simulink model "Pokus07_Display"  (Simulink 8.1)
settings: Solver=ode45  StartTime=0.0  StopTime=10.0  RelTol=1e-3
undefined symbols (not defined in the file): A, ARROW_DOWN, ARROW_LEFT, ARROW_RIGHT, ARROW_UP, ASTERISK, B, BACKSLASH, C, COLON, COMMA, CROSS, CURSOR, D, DOT, ending_column_index, ending_row_index, EQUAL, EXCLAMATION_MARK, F, framebuffer, G, GREATER_THAN, H, HEIGHT, hot, I, J, K, L, LEFT_PARENTHESES, LESS_THAN, M, MINUS, N, O, P, PERCENT, PLUS, POS_X, POS_Y, Q, QUESTION_MARK, QUOTE, R, RECTANGLE, RIGHT_PARENTHESES, S, SEMICOLON, SHARP, SLASH, SPACE, starting_column_index, starting_row_index, T, U, UNDERSCORE, V, W, WIDTH ... (+6)
libraries: dspmtrx3 x197, Common_Library x69, commutil2 x53, simulink_extras x1, dspsnks4 x1
(part 6 of 6)

== system Pokus07_Display/Character_Table/Characters(Q..ARROW_UP)/Char_GREATER_THAN ==
  Byte_01 : Constant  Value=char(:, 2, GREATER_THAN)  OutDataTypeStr=uint8
  Byte_02 : Constant  Value=char(:, 3, GREATER_THAN)  OutDataTypeStr=uint8
  Byte_03 : Constant  Value=char(:, 4, GREATER_THAN)  OutDataTypeStr=uint8
  Byte_04 : Constant  Value=char(:, 5, GREATER_THAN)  OutDataTypeStr=uint8
  Byte_05 : Constant  Value=char(:, 6, GREATER_THAN)  OutDataTypeStr=uint8
  Byte_06 : Constant  Value=char(:, 7, GREATER_THAN)  OutDataTypeStr=uint8
  Byte_07 : Constant  Value=char(:, 8, GREATER_THAN)  OutDataTypeStr=uint8
  Byte_1 : Constant  Value=char(:, 1, GREATER_THAN)  OutDataTypeStr=uint8
  Column_1(1B) : Outport
  Column_2(1B) : Outport  Port=2
  Column_3(1B) : Outport  Port=3
  Column_4(1B) : Outport  Port=4
  Column_5(1B) : Outport  Port=5
  Column_6(1B) : Outport  Port=6
  Column_7(1B) : Outport  Port=7
  Column_8(1B) : Outport  Port=8
  wires:
  Byte_05/1 -> Column_6(1B)/1
  Byte_04/1 -> Column_5(1B)/1
  Byte_01/1 -> Column_2(1B)/1
  Byte_07/1 -> Column_8(1B)/1
  Byte_03/1 -> Column_4(1B)/1
  Byte_06/1 -> Column_7(1B)/1
  Byte_1/1 -> Column_1(1B)/1
  Byte_02/1 -> Column_3(1B)/1

== system Pokus07_Display/Character_Table/Characters(Q..ARROW_UP)/Char_LESS_THAN ==
  Byte_01 : Constant  Value=char(:, 2, LESS_THAN)  OutDataTypeStr=uint8
  Byte_02 : Constant  Value=char(:, 3, LESS_THAN)  OutDataTypeStr=uint8
  Byte_03 : Constant  Value=char(:, 4, LESS_THAN)  OutDataTypeStr=uint8
  Byte_04 : Constant  Value=char(:, 5, LESS_THAN)  OutDataTypeStr=uint8
  Byte_05 : Constant  Value=char(:, 6, LESS_THAN)  OutDataTypeStr=uint8
  Byte_06 : Constant  Value=char(:, 7, LESS_THAN)  OutDataTypeStr=uint8
  Byte_07 : Constant  Value=char(:, 8, LESS_THAN)  OutDataTypeStr=uint8
  Byte_1 : Constant  Value=char(:, 1, LESS_THAN)  OutDataTypeStr=uint8
  Column_1(1B) : Outport
  Column_2(1B) : Outport  Port=2
  Column_3(1B) : Outport  Port=3
  Column_4(1B) : Outport  Port=4
  Column_5(1B) : Outport  Port=5
  Column_6(1B) : Outport  Port=6
  Column_7(1B) : Outport  Port=7
  Column_8(1B) : Outport  Port=8
  wires:
  Byte_05/1 -> Column_6(1B)/1
  Byte_04/1 -> Column_5(1B)/1
  Byte_01/1 -> Column_2(1B)/1
  Byte_07/1 -> Column_8(1B)/1
  Byte_03/1 -> Column_4(1B)/1
  Byte_06/1 -> Column_7(1B)/1
  Byte_1/1 -> Column_1(1B)/1
  Byte_02/1 -> Column_3(1B)/1

== system Pokus07_Display/Character_Table/Characters(Q..ARROW_UP)/Char_MINUS ==
  Byte_01 : Constant  Value=char(:, 2, MINUS)  OutDataTypeStr=uint8
  Byte_02 : Constant  Value=char(:, 3, MINUS)  OutDataTypeStr=uint8
  Byte_03 : Constant  Value=char(:, 4, MINUS)  OutDataTypeStr=uint8
  Byte_04 : Constant  Value=char(:, 5, MINUS)  OutDataTypeStr=uint8
  Byte_05 : Constant  Value=char(:, 6, MINUS)  OutDataTypeStr=uint8
  Byte_06 : Constant  Value=char(:, 7, MINUS)  OutDataTypeStr=uint8
  Byte_07 : Constant  Value=char(:, 8, MINUS)  OutDataTypeStr=uint8
  Byte_1 : Constant  Value=char(:, 1, MINUS)  OutDataTypeStr=uint8
  Column_1(1B) : Outport
  Column_2(1B) : Outport  Port=2
  Column_3(1B) : Outport  Port=3
  Column_4(1B) : Outport  Port=4
  Column_5(1B) : Outport  Port=5
  Column_6(1B) : Outport  Port=6
  Column_7(1B) : Outport  Port=7
  Column_8(1B) : Outport  Port=8
  wires:
  Byte_05/1 -> Column_6(1B)/1
  Byte_04/1 -> Column_5(1B)/1
  Byte_01/1 -> Column_2(1B)/1
  Byte_07/1 -> Column_8(1B)/1
  Byte_03/1 -> Column_4(1B)/1
  Byte_06/1 -> Column_7(1B)/1
  Byte_1/1 -> Column_1(1B)/1
  Byte_02/1 -> Column_3(1B)/1

== system Pokus07_Display/Character_Table/Characters(Q..ARROW_UP)/Char_PLUS ==
  Byte_01 : Constant  Value=char(:, 2, PLUS)  OutDataTypeStr=uint8
  Byte_02 : Constant  Value=char(:, 3, PLUS)  OutDataTypeStr=uint8
  Byte_03 : Constant  Value=char(:, 4, PLUS)  OutDataTypeStr=uint8
  Byte_04 : Constant  Value=char(:, 5, PLUS)  OutDataTypeStr=uint8
  Byte_05 : Constant  Value=char(:, 6, PLUS)  OutDataTypeStr=uint8
  Byte_06 : Constant  Value=char(:, 7, PLUS)  OutDataTypeStr=uint8
  Byte_07 : Constant  Value=char(:, 8, PLUS)  OutDataTypeStr=uint8
  Byte_1 : Constant  Value=char(:, 1, PLUS)  OutDataTypeStr=uint8
  Column_1(1B) : Outport
  Column_2(1B) : Outport  Port=2
  Column_3(1B) : Outport  Port=3
  Column_4(1B) : Outport  Port=4
  Column_5(1B) : Outport  Port=5
  Column_6(1B) : Outport  Port=6
  Column_7(1B) : Outport  Port=7
  Column_8(1B) : Outport  Port=8
  wires:
  Byte_05/1 -> Column_6(1B)/1
  Byte_04/1 -> Column_5(1B)/1
  Byte_01/1 -> Column_2(1B)/1
  Byte_07/1 -> Column_8(1B)/1
  Byte_03/1 -> Column_4(1B)/1
  Byte_06/1 -> Column_7(1B)/1
  Byte_1/1 -> Column_1(1B)/1
  Byte_02/1 -> Column_3(1B)/1

== system Pokus07_Display/Character_Table/Characters(Q..ARROW_UP)/Char_Q ==
  Byte_01 : Constant  Value=char(:, 2, Q)  OutDataTypeStr=uint8
  Byte_02 : Constant  Value=char(:, 3, Q)  OutDataTypeStr=uint8
  Byte_03 : Constant  Value=char(:, 4, Q)  OutDataTypeStr=uint8
  Byte_04 : Constant  Value=char(:, 5, Q)  OutDataTypeStr=uint8
  Byte_05 : Constant  Value=char(:, 6, Q)  OutDataTypeStr=uint8
  Byte_06 : Constant  Value=char(:, 7, Q)  OutDataTypeStr=uint8
  Byte_07 : Constant  Value=char(:, 8, Q)  OutDataTypeStr=uint8
  Byte_1 : Constant  Value=char(:, 1, Q)  OutDataTypeStr=uint8
  Column_1(1B) : Outport
  Column_2(1B) : Outport  Port=2
  Column_3(1B) : Outport  Port=3
  Column_4(1B) : Outport  Port=4
  Column_5(1B) : Outport  Port=5
  Column_6(1B) : Outport  Port=6
  Column_7(1B) : Outport  Port=7
  Column_8(1B) : Outport  Port=8
  wires:
  Byte_05/1 -> Column_6(1B)/1
  Byte_04/1 -> Column_5(1B)/1
  Byte_01/1 -> Column_2(1B)/1
  Byte_07/1 -> Column_8(1B)/1
  Byte_03/1 -> Column_4(1B)/1
  Byte_06/1 -> Column_7(1B)/1
  Byte_1/1 -> Column_1(1B)/1
  Byte_02/1 -> Column_3(1B)/1

== system Pokus07_Display/Character_Table/Characters(Q..ARROW_UP)/Char_SEMICOLON ==
  Byte_01 : Constant  Value=char(:, 2, SEMICOLON)  OutDataTypeStr=uint8
  Byte_02 : Constant  Value=char(:, 3, SEMICOLON)  OutDataTypeStr=uint8
  Byte_03 : Constant  Value=char(:, 4, SEMICOLON)  OutDataTypeStr=uint8
  Byte_04 : Constant  Value=char(:, 5, SEMICOLON)  OutDataTypeStr=uint8
  Byte_05 : Constant  Value=char(:, 6, SEMICOLON)  OutDataTypeStr=uint8
  Byte_06 : Constant  Value=char(:, 7, SEMICOLON)  OutDataTypeStr=uint8
  Byte_07 : Constant  Value=char(:, 8, SEMICOLON)  OutDataTypeStr=uint8
  Byte_1 : Constant  Value=char(:, 1, SEMICOLON)  OutDataTypeStr=uint8
  Column_1(1B) : Outport
  Column_2(1B) : Outport  Port=2
  Column_3(1B) : Outport  Port=3
  Column_4(1B) : Outport  Port=4
  Column_5(1B) : Outport  Port=5
  Column_6(1B) : Outport  Port=6
  Column_7(1B) : Outport  Port=7
  Column_8(1B) : Outport  Port=8
  wires:
  Byte_05/1 -> Column_6(1B)/1
  Byte_04/1 -> Column_5(1B)/1
  Byte_01/1 -> Column_2(1B)/1
  Byte_07/1 -> Column_8(1B)/1
  Byte_03/1 -> Column_4(1B)/1
  Byte_06/1 -> Column_7(1B)/1
  Byte_1/1 -> Column_1(1B)/1
  Byte_02/1 -> Column_3(1B)/1

== system Pokus07_Display/Character_Table/Characters(Q..ARROW_UP)/Char_SLASH ==
  Byte_01 : Constant  Value=char(:, 2, SLASH)  OutDataTypeStr=uint8
  Byte_02 : Constant  Value=char(:, 3, SLASH)  OutDataTypeStr=uint8
  Byte_03 : Constant  Value=char(:, 4, SLASH)  OutDataTypeStr=uint8
  Byte_04 : Constant  Value=char(:, 5, SLASH)  OutDataTypeStr=uint8
  Byte_05 : Constant  Value=char(:, 6, SLASH)  OutDataTypeStr=uint8
  Byte_06 : Constant  Value=char(:, 7, SLASH)  OutDataTypeStr=uint8
  Byte_07 : Constant  Value=char(:, 8, SLASH)  OutDataTypeStr=uint8
  Byte_1 : Constant  Value=char(:, 1, SLASH)  OutDataTypeStr=uint8
  Column_1(1B) : Outport
  Column_2(1B) : Outport  Port=2
  Column_3(1B) : Outport  Port=3
  Column_4(1B) : Outport  Port=4
  Column_5(1B) : Outport  Port=5
  Column_6(1B) : Outport  Port=6
  Column_7(1B) : Outport  Port=7
  Column_8(1B) : Outport  Port=8
  wires:
  Byte_05/1 -> Column_6(1B)/1
  Byte_04/1 -> Column_5(1B)/1
  Byte_01/1 -> Column_2(1B)/1
  Byte_07/1 -> Column_8(1B)/1
  Byte_03/1 -> Column_4(1B)/1
  Byte_06/1 -> Column_7(1B)/1
  Byte_1/1 -> Column_1(1B)/1
  Byte_02/1 -> Column_3(1B)/1

== system Pokus07_Display/Character_Table/Characters(Q..ARROW_UP)/Char_X ==
  Byte_01 : Constant  Value=char(:, 2, X)  OutDataTypeStr=uint8
  Byte_02 : Constant  Value=char(:, 3, X)  OutDataTypeStr=uint8
  Byte_03 : Constant  Value=char(:, 4, X)  OutDataTypeStr=uint8
  Byte_04 : Constant  Value=char(:, 5, X)  OutDataTypeStr=uint8
  Byte_05 : Constant  Value=char(:, 6, X)  OutDataTypeStr=uint8
  Byte_06 : Constant  Value=char(:, 7, X)  OutDataTypeStr=uint8
  Byte_07 : Constant  Value=char(:, 8, X)  OutDataTypeStr=uint8
  Byte_1 : Constant  Value=char(:, 1, X)  OutDataTypeStr=uint8
  Column_1(1B) : Outport
  Column_2(1B) : Outport  Port=2
  Column_3(1B) : Outport  Port=3
  Column_4(1B) : Outport  Port=4
  Column_5(1B) : Outport  Port=5
  Column_6(1B) : Outport  Port=6
  Column_7(1B) : Outport  Port=7
  Column_8(1B) : Outport  Port=8
  wires:
  Byte_05/1 -> Column_6(1B)/1
  Byte_04/1 -> Column_5(1B)/1
  Byte_01/1 -> Column_2(1B)/1
  Byte_07/1 -> Column_8(1B)/1
  Byte_03/1 -> Column_4(1B)/1
  Byte_06/1 -> Column_7(1B)/1
  Byte_1/1 -> Column_1(1B)/1
  Byte_02/1 -> Column_3(1B)/1

== system Pokus07_Display/Character_Table/Characters(Q..ARROW_UP)/Char_Y ==
  Byte_01 : Constant  Value=char(:, 2, Y)  OutDataTypeStr=uint8
  Byte_02 : Constant  Value=char(:, 3, Y)  OutDataTypeStr=uint8
  Byte_03 : Constant  Value=char(:, 4, Y)  OutDataTypeStr=uint8
  Byte_04 : Constant  Value=char(:, 5, Y)  OutDataTypeStr=uint8
  Byte_05 : Constant  Value=char(:, 6, Y)  OutDataTypeStr=uint8
  Byte_06 : Constant  Value=char(:, 7, Y)  OutDataTypeStr=uint8
  Byte_07 : Constant  Value=char(:, 8, Y)  OutDataTypeStr=uint8
  Byte_1 : Constant  Value=char(:, 1, Y)  OutDataTypeStr=uint8
  Column_1(1B) : Outport
  Column_2(1B) : Outport  Port=2
  Column_3(1B) : Outport  Port=3
  Column_4(1B) : Outport  Port=4
  Column_5(1B) : Outport  Port=5
  Column_6(1B) : Outport  Port=6
  Column_7(1B) : Outport  Port=7
  Column_8(1B) : Outport  Port=8
  wires:
  Byte_05/1 -> Column_6(1B)/1
  Byte_04/1 -> Column_5(1B)/1
  Byte_01/1 -> Column_2(1B)/1
  Byte_07/1 -> Column_8(1B)/1
  Byte_03/1 -> Column_4(1B)/1
  Byte_06/1 -> Column_7(1B)/1
  Byte_1/1 -> Column_1(1B)/1
  Byte_02/1 -> Column_3(1B)/1

== system Pokus07_Display/Character_Table/Characters(Q..ARROW_UP)/Char_Z ==
  Byte_01 : Constant  Value=char(:, 2, Z)  OutDataTypeStr=uint8
  Byte_02 : Constant  Value=char(:, 3, Z)  OutDataTypeStr=uint8
  Byte_03 : Constant  Value=char(:, 4, Z)  OutDataTypeStr=uint8
  Byte_04 : Constant  Value=char(:, 5, Z)  OutDataTypeStr=uint8
  Byte_05 : Constant  Value=char(:, 6, Z)  OutDataTypeStr=uint8
  Byte_06 : Constant  Value=char(:, 7, Z)  OutDataTypeStr=uint8
  Byte_07 : Constant  Value=char(:, 8, Z)  OutDataTypeStr=uint8
  Byte_1 : Constant  Value=char(:, 1, Z)  OutDataTypeStr=uint8
  Column_1(1B) : Outport
  Column_2(1B) : Outport  Port=2
  Column_3(1B) : Outport  Port=3
  Column_4(1B) : Outport  Port=4
  Column_5(1B) : Outport  Port=5
  Column_6(1B) : Outport  Port=6
  Column_7(1B) : Outport  Port=7
  Column_8(1B) : Outport  Port=8
  wires:
  Byte_05/1 -> Column_6(1B)/1
  Byte_04/1 -> Column_5(1B)/1
  Byte_01/1 -> Column_2(1B)/1
  Byte_07/1 -> Column_8(1B)/1
  Byte_03/1 -> Column_4(1B)/1
  Byte_06/1 -> Column_7(1B)/1
  Byte_1/1 -> Column_1(1B)/1
  Byte_02/1 -> Column_3(1B)/1
